simulink model "Microgrid_w_BESS_Q4_1"  (R2024b)
settings: Solver=VariableStepAuto  StartTime=0.0  StopTime=4  RelTol=1e-3
undefined symbols (not defined in the file): DiscIntNeverNeededParam, ini_SoC, Ion, Lithium, Ts, Ts_Control
libraries: simulink x5, ee_lib x5, spsParallelRLCBranchLib x4, nesl_utility x4, spsCurrentVoltageSimscapeInterfaceLib x3, powerlib_extras x3, spsThreePhaseVIMeasurementLib x2, spsSeriesRLCBranchLib x2, spsMultimeterLib x2, spsThreePhaseSeriesRLCBranchLib x2, spsGroundLib x2, slpidlib x2
(part 1 of 2)
settings Model: Creator=DELL  LastModifiedBy=mitphanase
settings DataIOCC: ReturnWorkspaceOutputs=off

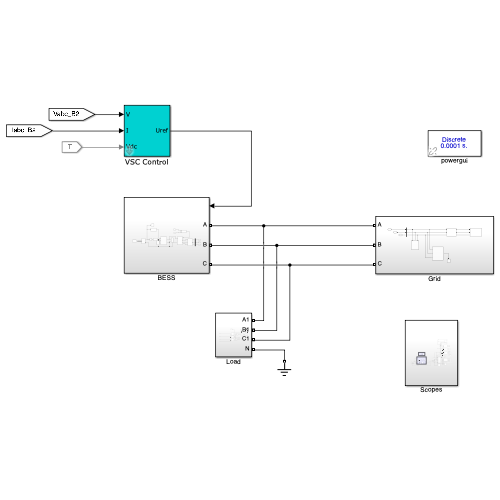
[thumbnail: Simulink's stored preview of the top-level diagram]
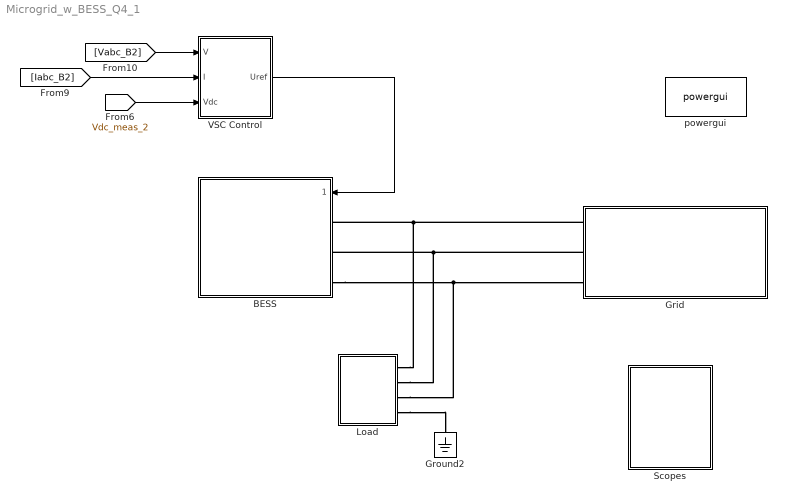
== system Microgrid_w_BESS_Q4_1 ==
  BESS : Subsystem
  Grid : Subsystem
  Ground2 : spsGroundLib/Ground  LConnTagsString=a
  Load : Subsystem
  Scopes : Subsystem
  VSC Control : Subsystem  mask(VSC Main Controller){nom=[10e3  50 ], Vnom=[ 400 400 ], Vnom_dc=600, RLxfo=[0  0 ], RLchoke=[0  0  ], K_VDCreg=[18  600], K_Ireg=[0.2 20], Ts=Ts_Control}
      mask prompts: nom "Nominal power and frequency [ Pnom(VA)  Fnom(Hz) ]:"; Vnom "Nominal primary and secondary voltages (Vrms LL) [ Vnom_prim   Vnom_sec ]:"; Vnom_dc "Nominal DC bus voltage (V):"; RLxfo "Total transformer leakage impedance (pu/Pnom) [ Rxfo  Lxf ]"; RLchoke "Choke impedance [ R(ohm) L(H) ]"; K_VDCreg "VDC regultator gains [ Kp  Ki ]:"; K_Ireg "Current regulator gains [ Kp  Ki ]:"; Ts "Sample time"
      mask init:
      | Pnom=nom(1);
      | Fnom=nom(2);
      | Vnom_prim=Vnom(1);
      | Vnom_sec=Vnom(2);
      | Zbase=Vnom_sec^2/Pnom;
      | Rtot_pu=RLxfo(1) + RLchoke(1)/Zbase;
      | Ltot_pu=RLxfo(2) + RLchoke(2)/(Zbase/(2*pi*Fnom));
      | Kp_VDCreg=K_VDCreg(1);
      | Ki_VDCreg=K_VDCreg(2);
      | Kp_Ireg=K_Ireg(1);
      | Ki_Ireg=K_Ireg(2);
      | Vdc_ref=Vnom_dc;
  powergui : sps_lib/powergui  Priority=1  SimulationMode=Discrete  SampleTime=Ts  frequency=60  Iterations=50  frequencyindice=0  Pbase=100e6  ErrMax=1e-4  UnitsV=kV  UnitsW=MW  buscounter=0  FunctionMessages=off  echomessages=off  EnableUseOfTLC=off  CurrentSourceSwitches=off  DisableSnubberDevices=off  DisableRonSwitches=off  DisableVfSwitches=off  DisplayEquations=off  AutomaticDiscreteSolvers=off  SolverType=Tustin/Backward Euler (TBE)  Interpol=off  ExternalGateDelay=off  methode=off  Ts=100  x0status=blocks  SPID=on  SwTol=0  HookPort=off  NonlinearTolerance=1e-4  nMaxIteration=100  ContinueOnMaxIteration=off  RestoreLinks=warning  ResistiveCurrentMeasurement=off  Frange=[0:2:500]  Ylog=off  Xlog=on  ShowGrid=off  save=off  variable=ZData  structure=0  ZoomFFT=off  StartTime=0.0  cycles=1  DisplayStyle=1  fundamental=60  FreqAxis=off  MaxFrequency=1000  frequencyindicesteady=1  RmsSteady=1  display=off
  wires:
  [Vdc_meas_2] -> VSC Control/3(Vdc)
  [Vabc_B2] -> VSC Control/1(V)
  [Iabc_B2] -> VSC Control/2(I)
  VSC Control/1(Uref) -> BESS/1("  ")
  connections:
  Grid/LConn1 -- Load/LConn1 -- BESS/LConn1
  BESS/LConn3 -- Load/LConn3 -- Grid/LConn3
  Grid/LConn2 -- Load/LConn2 -- BESS/LConn2
  Load/LConn4 -- Ground2/LConn1

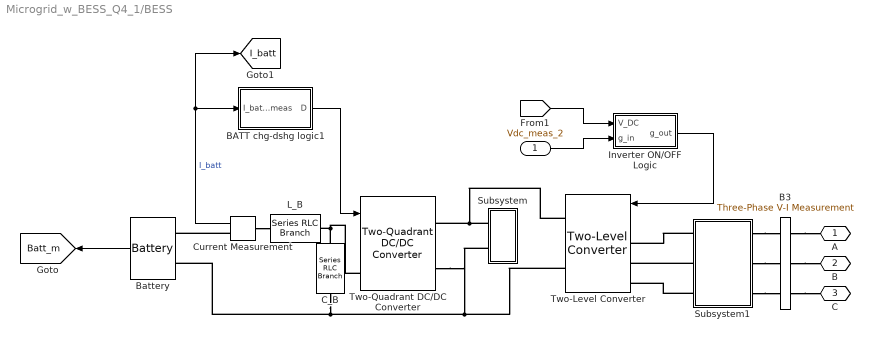
== system Microgrid_w_BESS_Q4_1/BESS ==
  "  " : Inport
  B3 : spsThreePhaseVIMeasurementLib/Three-Phase V-I Measurement  VoltageMeasurement=phase-to-ground  SetLabelV=on  LabelV=Vabc_B3  Vpu=off  VpuLL=off  CurrentMeasurement=yes  SetLabelI=on  LabelI=Iabc_B3  Ipu=off  Pbase=100e6  Vbase=1000  OutputType=Magnitude  PhasorSimulation=off  PSBequivalent=0
  BATT chg-dshg logic1 : Subsystem
  Battery : spsBatteryLib/Battery  BatType=Lithium-Ion  NomV=500  NomQ=20  SOC=ini_SoC  Batt_Tr=0.01  PresetModel=on  MaxQ=20  MinV=375  FullV=581.9936  Dis_rate=8.6957  R=0.25  Normal_OP=18.087  expZone="[540.1929     0.9826087]"
  C_B : spsSeriesRLCBranchLib/Series RLC Branch  LConnTagsString=__new0  RConnTagsString=__new0  BranchType=C  Resistance=10e-3  Inductance=10e-3  SetiL0=off  InitialCurrent=0  Capacitance=100e-6  Setx0=off  InitialVoltage=230  Measurements=None
  Current Measurement : spsCurrentMeasurementLib/Current Measurement  PhasorSimulation=off  OutputType=Complex  PSBequivalent=0
  Inverter ON/OFF Logic : Subsystem
  L_B : spsSeriesRLCBranchLib/Series RLC Branch  LConnTagsString=__new0  RConnTagsString=__new0  BranchType=RL  Resistance=0.5  Inductance=10e-3  SetiL0=off  InitialCurrent=0  Capacitance=100e-6  Setx0=off  InitialVoltage=230  Measurements=None
  Subsystem : Subsystem
  Subsystem1 : Subsystem
  Two-Level Converter : spsTwoLevelConverterLib/Two-Level Converter  ModelType=Average model (Uref-controlled)  Ron=1e-3  Rs=1e6  Cs=inf  Vforward=[0,0]  Ron_Diode=1e-3  Rs_Diode=1e6  Cs_Diode=inf  Vf_Diode=1e-3  Rs_CurrentSource=inf  Ron_ACsource=1e-3
      settings: LibrarySourceBlock=sps_lib/Power Electronics/Two-Level Converter
  Two-Quadrant DC/DC Converter : spsTwoQuadrantDCDCConverterLib/Two-Quadrant DC//DC Converter  ModelType=Average model (D-controlled)  Ron=1e-3  Rs=1e6  Cs=inf  Vforward=[0,0]  Ron_Diode=1e-3  Rs_Diode=1e6  Cs_Diode=inf  Vf_Diode=1e-3  Rs_CurrentSource=inf  Ron_ACsource=1e-3
  A : PMIOPort  Side=Left
  B : PMIOPort  Port=2  Side=Left
  C : PMIOPort  Port=3  Side=Left
  tag scope: Batt_m=global, I_batt=global
  wires:
  BATT chg-dshg logic1/1(D) -> Two-Quadrant DC/DC Converter/1
  [Vdc_meas_2] -> Inverter ON/OFF Logic/1(V_DC)
  "  "/1 -> Inverter ON/OFF Logic/2(g_in)
  Inverter ON/OFF Logic/1(g_out) -> Two-Level Converter/1
  Battery/1 -> [Batt_m]
  Current Measurement/1 -> BATT chg-dshg logic1/1(I_batt_meas), [I_batt]  "I_batt"
  connections:
  Two-Level Converter/RConn2 -- Subsystem/RConn2 -- Two-Quadrant DC/DC Converter/RConn2 -- Battery/LConn2 -- C_B/RConn1
  C_B/LConn1 -- Two-Quadrant DC/DC Converter/LConn1 -- L_B/LConn1
  Subsystem/RConn1 -- Two-Level Converter/RConn1 -- Two-Quadrant DC/DC Converter/RConn1
  Current Measurement/LConn1 -- L_B/RConn1
  Current Measurement/RConn1 -- Battery/LConn1
  B3/RConn1 -- A/RConn1
  B3/RConn2 -- B/RConn1
  B3/RConn3 -- C/RConn1
  Subsystem1/RConn1 -- B3/LConn1
  Subsystem1/RConn2 -- B3/LConn2
  Subsystem1/RConn3 -- B3/LConn3
  Subsystem1/LConn2 -- Two-Level Converter/LConn2
  Subsystem1/LConn1 -- Two-Level Converter/LConn1
  Subsystem1/LConn3 -- Two-Level Converter/LConn3

== system Microgrid_w_BESS_Q4_1/Grid ==
  B2 : spsThreePhaseVIMeasurementLib/Three-Phase V-I Measurement  VoltageMeasurement=phase-to-ground  SetLabelV=on  LabelV=Vabc_B2  Vpu=off  VpuLL=off  CurrentMeasurement=yes  SetLabelI=on  LabelI=Iabc_B2  Ipu=off  Pbase=100e6  Vbase=500e3  OutputType=Magnitude  PhasorSimulation=off  PSBequivalent=0
  Ground : spsGroundLib/Ground  LConnTagsString=a
  "Grounding Transformer " : spsGroundingTransformerLib/Grounding Transformer   UNITS=SI  NominalPower="[3e3   50]"  NominalVoltage=0.4e3  ZeroSequenceImpedance_pu=[0.025 0.75]  MagnetizationBranch_pu=[500 500]  ZeroSequenceImpedance_SI=[1.3333 40]  MagnetizationBranch_SI=[26667 26667]  Measurements=All voltages and currents
      settings: LibrarySourceBlock=|
      | sps_lib/Power Grid Elements/Grounding
      | Transformer
  Three-Phase Series RLC Branch : spsThreePhaseSeriesRLCBranchLib/Three-Phase Series RLC Branch  LConnTagsString=A|B|C  RConnTagsString=A|B|C  BranchType=R  Resistance=1e-3  Inductance=1e-3  Capacitance=1e-6  Measurements=None
  Three-Phase Series RLC Load1 : spsThreePhaseSeriesRLCLoadLib/Three-Phase Series RLC Load  LConnTagsString=A|B|C  Configuration=Y (grounded)  NominalVoltage=400  Vabc=[1e3 1e3 1e3]  Vabcp=[1e3 1e3 1e3]  NominalFrequency=50  UnbalancedPower=off  ActivePower=1  InductivePower=0  CapacitivePower=0  Pabc=[10e3 9e3 11e3]  QLabc=[100 90 110]  QCabc=[100 90 110]  Pabcp=[10e3 9e3 11e3]  QLabcp=[100 90 110]  QCabcp=[100 90 110]  Measurements=None  LoadType=constant Z
  Three-Phase Source : spsThreePhaseSourceLib/Three-Phase Source  InternalConnection=Yg  VoltagePhases=off  Voltage=400  PhaseAngle=0  Voltage_phases=[25e3 25e3 25e3]/sqrt(3)  PhaseAngles_phases=[0 -120 +120]  Frequency=50  NonIdealSource=on  SpecifyImpedance=on  Resistance=0.0113  Inductance=36e-6  ShortCircuitLevel=1e6  BaseVoltage=400  XRratio=4  BusType=swing  Pref=10e3  Qref=0  Prefabc=[10e3, 10e3, 10e3]  Qrefabc=[0, 0, 0]  Qmin=-inf  Qmax=inf
  A : PMIOPort  Side=Left
  B : PMIOPort  Port=2  Side=Left
  C : PMIOPort  Port=3  Side=Left
  connections:
  "Grounding Transformer "/RConn1 -- Ground/LConn1
  B2/LConn1 -- Three-Phase Series RLC Branch/LConn1 -- "Grounding Transformer "/LConn1 -- Three-Phase Series RLC Load1/LConn1
  Three-Phase Series RLC Load1/LConn2 -- Three-Phase Series RLC Branch/LConn2 -- "Grounding Transformer "/LConn2 -- B2/LConn2
  Three-Phase Series RLC Load1/LConn3 -- Three-Phase Series RLC Branch/LConn3 -- "Grounding Transformer "/LConn3 -- B2/LConn3
  B2/RConn3 -- C/RConn1
  B2/RConn2 -- B/RConn1
  B2/RConn1 -- A/RConn1
  Three-Phase Series RLC Branch/RConn1 -- Three-Phase Source/RConn1
  Three-Phase Series RLC Branch/RConn2 -- Three-Phase Source/RConn2
  Three-Phase Series RLC Branch/RConn3 -- Three-Phase Source/RConn3

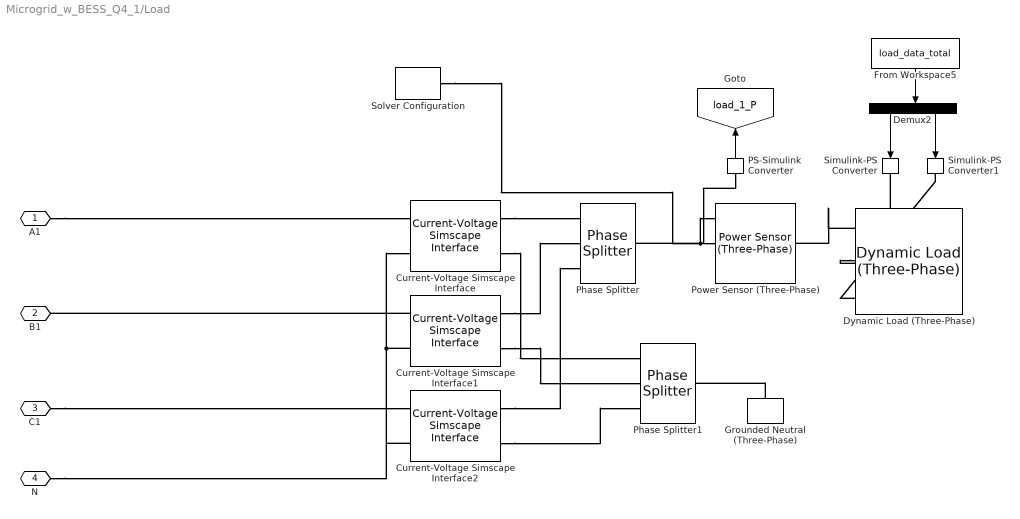
== system Microgrid_w_BESS_Q4_1/Load ==
  Current-Voltage Simscape Interface : spsCurrentVoltageSimscapeInterfaceLib/Current-Voltage Simscape Interface  DFT=off  FMode=Low pass filter (continuous)  T=1e-4  Ts=50e-6  i0=0  v0=0  Sd=Specialized Power Systems side  Measurements=off
  Current-Voltage Simscape Interface1 : spsCurrentVoltageSimscapeInterfaceLib/Current-Voltage Simscape Interface  DFT=off  FMode=Low pass filter (continuous)  T=1e-4  Ts=50e-6  i0=0  v0=0  Sd=Specialized Power Systems side  Measurements=off
  Current-Voltage Simscape Interface2 : spsCurrentVoltageSimscapeInterfaceLib/Current-Voltage Simscape Interface  DFT=off  FMode=Low pass filter (continuous)  T=1e-4  Ts=50e-6  i0=0  v0=0  Sd=Specialized Power Systems side  Measurements=off
  Demux2 : Demux  Outputs=2
  Dynamic Load (Three-Phase) : ee_lib/Passive/Dynamic Load (Three-Phase)  port_option=ee.enum.threePhasePort.composite  FRated=50 Hz  Vline_rms_min=1 V  tau=0.01 s  Vline_rms_ini=400 V  Vang_ini=0 deg  gmin=0 S  fault_action=simscape.enum.assert.action.none  t_fault=1 s
      settings: InternalSimscapePortConfiguration="{\"Bottom\":[],\"Left\":[{\"id\":\"N\",\"label\":\"~\",\"type\":\"foundation.electrical.three_phase\"}],\"Right\":[],\"Top\":[{\"id\":\"P\",\"label\":\"P\",\"type\":\"input\"},{\"id\":\"Q\",\"label\":\"Q\",\"type\":\"input\"}]}"
  From Workspace5 : FromWorkspace  VariableName=load_data_total  SampleTime=0.01
  Grounded Neutral (Three-Phase) : ee_lib/Connectors & References/Grounded Neutral (Three-Phase)
  PS-Simulink Converter : nesl_utility/PS-Simulink Converter  PhysicalDomain=network_engine_domain  SubClassName=ps_output  LeftPortType=input  RightPortType=output  PseudoPeriodic=off  Frequencies=[]  VectorFormat=inherit  Unit=inherit  AffineConversion=off
  Phase Splitter : ee_lib/Connectors & References/Phase Splitter
  Phase Splitter1 : ee_lib/Connectors & References/Phase Splitter
  Power Sensor (Three-Phase) : ee_lib/Sensors & Transducers/Power Sensor (Three-Phase)  load_type=ee.enum.passive.type_balanced.unbalanced  f0=50 Hz  config=ee.enum.with_neutral.no  rho=1
      settings: InternalSimscapePortConfiguration="{\"Bottom\":[],\"Left\":[{\"id\":\"N1\",\"label\":\"~1\",\"type\":\"foundation.electrical.three_phase\"}],\"Right\":[{\"id\":\"N2\",\"label\":\"~2\",\"type\":\"foundation.electrical.three_phase\"}],\"Top\":[{\"id\":\"Pm\",\"label\":\"P\",\"type\":\"output\"},{\"id\":\"Qm\",\"label\":\"Q\",\"type\":\"output\"}]}"
  Simulink-PS Converter : nesl_utility/Simulink-PS Converter  PhysicalDomain=network_engine_domain  SubClassName=ps_input  LeftPortType=input  RightPortType=output  PseudoPeriodic=off  Frequencies=[]  NoiseDistribution=none  NoiseParameters=[]  Unit=1  AffineConversion=off  FilteringAndDerivatives=provide  SimscapeFilterOrder=1  InputFilterTimeConstant=0.001  UdotUserProvided=0
  Simulink-PS Converter1 : nesl_utility/Simulink-PS Converter  PhysicalDomain=network_engine_domain  SubClassName=ps_input  LeftPortType=input  RightPortType=output  PseudoPeriodic=off  Frequencies=[]  NoiseDistribution=none  NoiseParameters=[]  Unit=1  AffineConversion=off  FilteringAndDerivatives=provide  SimscapeFilterOrder=1  InputFilterTimeConstant=0.001  UdotUserProvided=0
  Solver Configuration : nesl_utility/Solver Configuration  PhysicalDomain=network_engine_domain  SubClassName=solver  LeftPortType=input  RightPortType=generic  Tones=[]  Harmonics=[]  SimulateNoise=off  Profile=off  UseLocalSampling=off  EnableSwitchedLinearOptims=on  FrequencyDomain=off  UseCCode=off  RelTol=0.001  AbsTol=0.001  MinStep=1e-09  ToWorkspace=off  RevertToSquareIcSolve=off  NumHomotopyIterations=100  PhasorMode=off  PhasorModeNumHarmonics=1  ConsistencySolver=NEWTON_XTOL_AFTER_FTOL  IndexReductionMethod=DerivativeReplacement  DoDC=on  ResidualTolerance=1e-09  ConsistencyTolSource=GLOBAL  ConsistencyAbsTol=0.001  ConsistencyRelTol=0.001  ConsistencyTolFactor=0.001  UseLocalSolver=off  LocalSolverChoice=NE_BACKWARD_EULER_ADVANCER  ResolveIndetEquations=on  FunctionEvalNumThread=1  LocalSolverSampleTime=0.0001  DoFixedCost=off  MaxNonlinIter=3  MaxModeIter=2  ComputeImpulses=off  ImpulseIterations=2  LinearAlgebra=Sparse  LinearAlgebraNumThread=0  EquationFormulation=NE_TIME_EF  DelaysMemoryBudget=2048  AutomaticFiltering=off  FilteringTimeConstant=0.001  PartitionStorageMethod=AS_NEEDED  PartitionMemoryBudget=1024  PartitionMethod=ROBUST  MultibodyUseLocalSolver=off  MultibodyLocalSolverChoice=ODE1  MultibodyLocalSolverSampleTime=0.001
  A1 : PMIOPort  Side=Left
  B1 : PMIOPort  Port=2  Side=Left
  C1 : PMIOPort  Port=3  Side=Left
  N : PMIOPort  Port=4  Side=Left
  tag scope: load_1_P=global
  wires:
  From Workspace5/1 -> Demux2/1
  Demux2/2 -> Simulink-PS Converter1/1
  PS-Simulink Converter/1 -> [load_1_P]
  Demux2/1 -> Simulink-PS Converter/1
  connections:
  Power Sensor (Three-Phase)/LConn1 -- Solver Configuration/RConn1 -- Phase Splitter/LConn1
  Current-Voltage Simscape Interface1/RConn2 -- Phase Splitter1/RConn2
  Current-Voltage Simscape Interface2/RConn2 -- Phase Splitter1/RConn3
  Dynamic Load (Three-Phase)/LConn1 -- Power Sensor (Three-Phase)/RConn1
  Current-Voltage Simscape Interface1/RConn1 -- Phase Splitter/RConn2
  Current-Voltage Simscape Interface2/RConn1 -- Phase Splitter/RConn3
  Current-Voltage Simscape Interface/RConn1 -- Phase Splitter/RConn1
  Dynamic Load (Three-Phase)/LConn3 -- Simulink-PS Converter1/RConn1
  Grounded Neutral (Three-Phase)/LConn1 -- Phase Splitter1/LConn1
  Current-Voltage Simscape Interface/RConn2 -- Phase Splitter1/RConn1
  PS-Simulink Converter/LConn1 -- Power Sensor (Three-Phase)/LConn2
  Dynamic Load (Three-Phase)/LConn2 -- Simulink-PS Converter/RConn1
  A1/RConn1 -- Current-Voltage Simscape Interface/LConn1
  Current-Voltage Simscape Interface1/LConn1 -- B1/RConn1
  Current-Voltage Simscape Interface1/LConn2 -- N/RConn1 -- Current-Voltage Simscape Interface2/LConn2 -- Current-Voltage Simscape Interface/LConn2
  C1/RConn1 -- Current-Voltage Simscape Interface2/LConn1

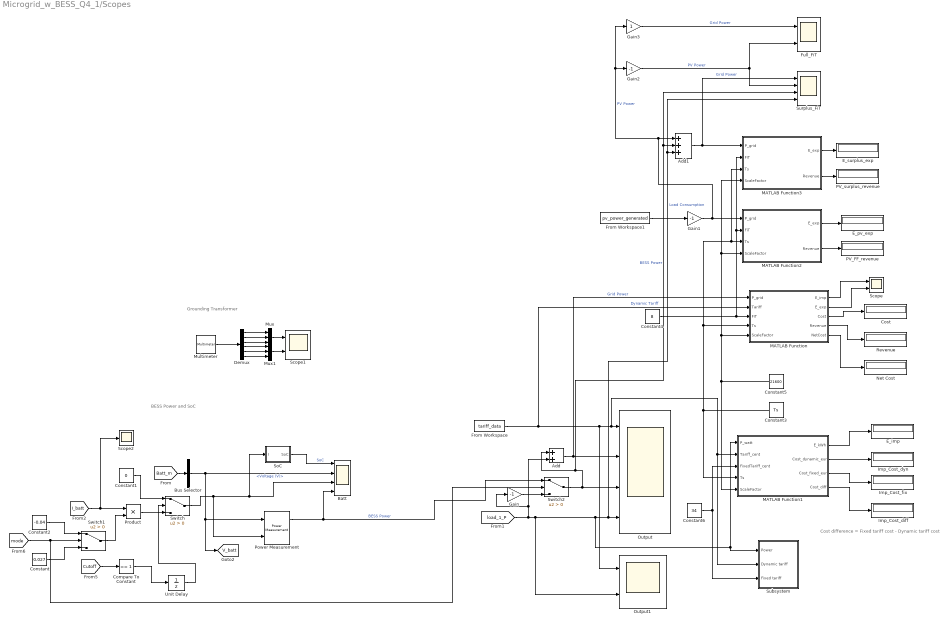
== system Microgrid_w_BESS_Q4_1/Scopes ==
  note: Cost difference = Fixed tariff cost - Dynamic tariff cost
  note: Grounding Transformer
  note: BESS Power and SoC
  Add : Sum
  Add1 : Sum  Inputs=+++
  Batt : Scope  NumInputPorts=4
  Bus Selector : BusSelector  OutputSignals=Voltage (V)
  Compare To Constant : simulink/Logic and Bit Operations/Compare To Constant  relop===  const=1  OutDataTypeStr=uint8
  Constant : Constant  Value=0.027
  Constant1 : Constant  Value=0
  Constant2 : Constant  Value=-0.04
  Constant3 : Constant  Value=Ts
  Constant4 : Constant  Value=8
  Constant5 : Constant  Value=21600
  Constant6 : Constant  Value=34
  Cost : Display
  Demux : Demux  Outputs=6
  E_imp : Display
  E_pv_exp : Display
  E_surplus_exp : Display
  From Workspace : FromWorkspace  VariableName=tariff_data  SampleTime=0.01
  From Workspace1 : FromWorkspace  VariableName=pv_power_generated
  Full_FiT : Scope  NumInputPorts=2
  Gain : Gain  Gain=-1
  Gain1 : Gain  Gain=-1
  Gain2 : Gain  Gain=-1
  Gain3 : Gain
  Imp_Cost_diff : Display
  Imp_Cost_dyn : Display
  Imp_Cost_fix : Display
  MATLAB Function : MATLAB Function  TreatAsAtomicUnit=on
  MATLAB Function1 : MATLAB Function  TreatAsAtomicUnit=on
  MATLAB Function2 : MATLAB Function  TreatAsAtomicUnit=on
  MATLAB Function3 : MATLAB Function  TreatAsAtomicUnit=on
  Multimeter : spsMultimeterLib/Multimeter  L=12  sel=[1 2 3 10 11 12]  yselected={}  Gain=[1 1 1 1 1 1]  OutputType=Complex  PlotAtSimulationStop=off  PhasorSimulation=off
  Mux : Mux  Inputs=3
  Mux1 : Mux  Inputs=3
  Net Cost : Display
  Output : Scope  NumInputPorts=4
  Output1 : Scope  NumInputPorts=2
  PV_FF_revenue : Display
  PV_surplus_revenue : Display
  Power Measurement : eePowerMeasurement/Power Measurement  LabelModeActiveChoice=Discrete  F=50  K=[0]  Ts=Ts_Control
  Product : Product
  Revenue : Display
  Scope : Scope  NumInputPorts=2
  Scope1 : Scope  NumInputPorts=2
  Scope2 : Scope
  SoC : Subsystem
  Subsystem : Subsystem
  Surplus_FiT : Scope  NumInputPorts=4
  Switch : Switch  Criteria=u2 > Threshold  SaturateOnIntegerOverflow=off  InputSameDT=off
  Switch1 : Switch  Criteria=u2 > Threshold  SaturateOnIntegerOverflow=off  InputSameDT=off
  Switch2 : Switch  Criteria=u2 > Threshold  SaturateOnIntegerOverflow=off  InputSameDT=off
  Unit Delay : UnitDelay  SampleTime=-1  HasFrameUpgradeWarning=on
  tag scope: V_batt=global
  wires:
  SoC/1(SoC) -> Batt/1  "SoC"
  [Batt_m] -> Bus Selector/1
  [load_1_P] -> Add/2, Gain/1, Output1/2, MATLAB Function1/1(P_watt), Subsystem/1(Power), Add1/3, Surplus_FiT/4, Output/4  "Load Consumption"
  Multimeter/1 -> Demux/1
  Demux/1 -> Mux/1
  Demux/2 -> Mux/2
  Mux/1 -> Scope1/1
  Demux/3 -> Mux/3
  Demux/4 -> Mux1/1
  Demux/5 -> Mux1/2
  Demux/6 -> Mux1/3
  Mux1/1 -> Scope1/2
  Bus Selector/1 -> Batt/2, Power Measurement/1, [V_batt]  "<Voltage (V)>"
  [I_batt] -> Scope2/1, Product/1
  Switch/1 -> SoC/1(I), Batt/3, Power Measurement/2
  [Cutoff] -> Compare To Constant/1
  Product/1 -> Switch/3
  Constant1/1 -> Switch/1
  Constant2/1 -> Switch1/1
  Constant/1 -> Switch1/3
  Switch1/1 -> Product/2
  [mode] -> Switch2/2, Switch1/2
  Compare To Constant/1 -> Unit Delay/1
  Unit Delay/1 -> Switch/2
  Power Measurement/1 -> Batt/4, Switch2/1  "BESS Power"
  From Workspace/1 -> MATLAB Function/2(Tariff), Output1/1, Subsystem/2(Dynamic tariff), MATLAB Function1/2(Tariff_cent), Output/1  "Dynamic Tariff"
  Add/1 -> MATLAB Function/1(P_grid), Output/2  "Grid Power"
  Constant3/1 -> MATLAB Function3/3(Ts), MATLAB Function2/3(Ts), MATLAB Function/4(Ts), MATLAB Function1/4(Ts)
  MATLAB Function/3(Cost) -> Cost/1
  MATLAB Function/1(E_imp) -> Scope/1
  MATLAB Function/2(E_exp) -> Scope/2
  Constant4/1 -> MATLAB Function3/2(FiT), MATLAB Function2/2(FiT), MATLAB Function/3(FiT)
  MATLAB Function/4(Revenue) -> Revenue/1
  MATLAB Function/5(NetCost) -> Net Cost/1
  Switch2/1 -> Add1/2, Surplus_FiT/3, Add/1, Output/3  "BESS Power"
  Gain/1 -> Switch2/3
  Constant5/1 -> MATLAB Function1/5(ScaleFactor), MATLAB Function3/4(ScaleFactor), MATLAB Function2/4(ScaleFactor), MATLAB Function/5(ScaleFactor)
  MATLAB Function1/1(E_kWh) -> E_imp/1
  MATLAB Function1/2(Cost_dynamic_eur) -> Imp_Cost_dyn/1
  Constant6/1 -> Subsystem/3(Fixed tariff), MATLAB Function1/3(FixedTariff_cent)
  MATLAB Function1/4(Cost_diff) -> Imp_Cost_diff/1
  MATLAB Function1/3(Cost_fixed_eur) -> Imp_Cost_fix/1
  MATLAB Function2/1(E_exp) -> E_pv_exp/1
  MATLAB Function2/2(Revenue) -> PV_FF_revenue/1
  Gain1/1 -> Gain3/1, Gain2/1, Add1/1, MATLAB Function2/1(P_grid)  "PV Power"
  From Workspace1/1 -> Gain1/1
  Add1/1 -> Surplus_FiT/1, MATLAB Function3/1(P_grid)  "Grid Power"
  MATLAB Function3/1(E_exp) -> E_surplus_exp/1
  MATLAB Function3/2(Revenue) -> PV_surplus_revenue/1
  Gain2/1 -> Full_FiT/2, Surplus_FiT/2  "PV Power"
  Gain3/1 -> Full_FiT/1  "Grid Power"

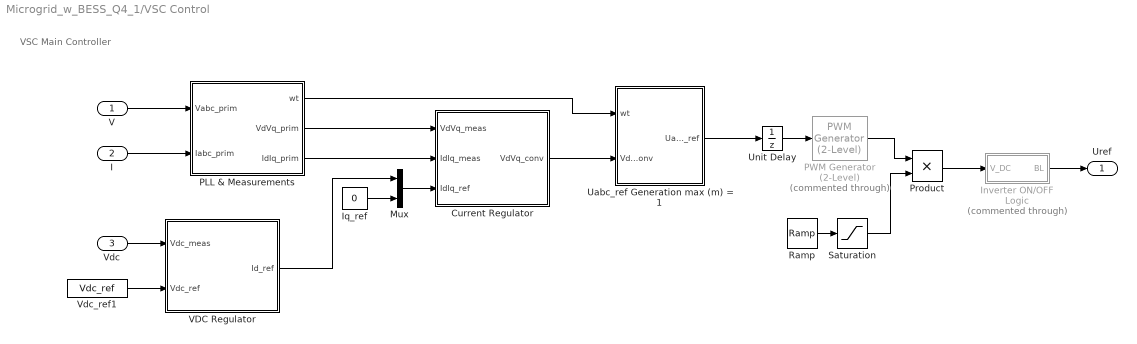
== system Microgrid_w_BESS_Q4_1/VSC Control ==
  note: VSC Main Controller
  V : Inport  PortDimensions=3
  I : Inport  Port=2  PortDimensions=3
  Vdc : Inport  Port=3  PortDimensions=1
  Current Regulator : Subsystem
  Inverter ON/OFF Logic : Subsystem  Commented=through
  Iq_ref : Constant  Value=0
  Mux : Mux  Inputs=2
  PLL & Measurements : Subsystem
  PWM Generator (2-Level) : spsPWMGenerator2LevelLib/PWM Generator (2-Level)  Commented=through  ModulatorType=Three-phase bridge (6 pulses)  ModulatorMode=Unsynchronized  Fc=27*50*8  Pc=90  nF=27  MinMax="[ -1  1 ]"  SamplingTechnique=Natural  ModulatingSignals=off  m=0.8  Freq=60  Phase=0  Ts=Ts_Control  ShowCarrierOutport=off
  Product : Product
  Ramp : simulink/Sources/Ramp  slope=1/0.02  start=0  InitialOutput=0
  Saturation : Saturate  UpperLimit=1  LowerLimit=0
  Uabc_ref Generation max (m) = 1 : Subsystem
  Unit Delay : UnitDelay  SampleTime=Ts_Control  HasFrameUpgradeWarning=on
  VDC Regulator : Subsystem
  Vdc_ref1 : Constant  Value=Vdc_ref
  Uref : Outport  VectorParamsAs1DForOutWhenUnconnected=off
  wires:
  Vdc_ref1/1 -> VDC Regulator/2(Vdc_ref)
  Uabc_ref Generation max (m) = 1/1(Uabc_ref) -> Unit Delay/1
  Unit Delay/1 -> PWM Generator (2-Level)/1
  I/1 -> PLL & Measurements/2(Iabc_prim)
  V/1 -> PLL & Measurements/1(Vabc_prim)
  Vdc/1 -> VDC Regulator/1(Vdc_meas)
  PLL & Measurements/2(VdVq_prim) -> Current Regulator/1(VdVq_meas)
  PLL & Measurements/3(IdIq_prim) -> Current Regulator/2(IdIq_meas)
  Mux/1 -> Current Regulator/3(IdIq_ref)
  Iq_ref/1 -> Mux/2
  PLL & Measurements/1(wt) -> Uabc_ref Generation max (m) = 1/1(wt)
  VDC Regulator/1(Id_ref) -> Mux/1
  PWM Generator (2-Level)/1 -> Product/1
  Current Regulator/1(VdVq_conv) -> Uabc_ref Generation max (m) = 1/2(VdVq_conv)
  Product/1 -> Inverter ON/OFF Logic/1(V_DC)
  Ramp/1 -> Saturation/1
  Saturation/1 -> Product/2
  Inverter ON/OFF Logic/1(BL) -> Uref/1

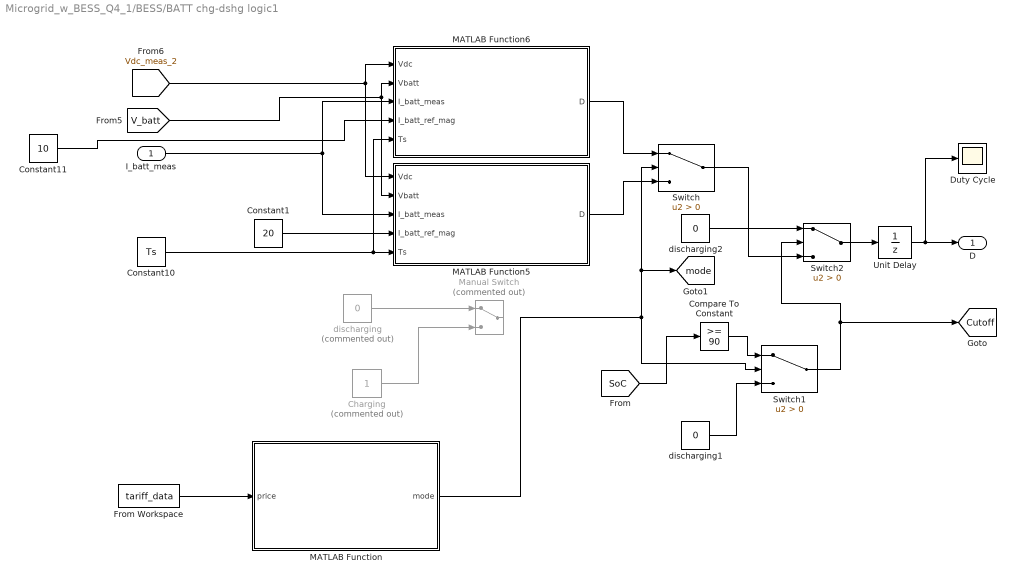
== system Microgrid_w_BESS_Q4_1/BESS/BATT chg-dshg logic1 ==
  I_batt_meas : Inport
  Charging : Constant  Commented=on
  Compare To Constant : simulink/Logic and Bit Operations/Compare To Constant  relop=>=  const=90  OutDataTypeStr=boolean
  Constant1 : Constant  Value=20
  Constant10 : Constant  Value=Ts
  Constant11 : Constant  Value=10
  Duty Cycle : Scope
  From Workspace : FromWorkspace  VariableName=tariff_data  SampleTime=0.01
  MATLAB Function : MATLAB Function  TreatAsAtomicUnit=on
  MATLAB Function5 : MATLAB Function  TreatAsAtomicUnit=on
  MATLAB Function6 : MATLAB Function  TreatAsAtomicUnit=on
  Manual Switch : ManualSwitch  Commented=on
  Switch : Switch  Criteria=u2 > Threshold  SaturateOnIntegerOverflow=off  InputSameDT=off
  Switch1 : Switch  Criteria=u2 > Threshold  SaturateOnIntegerOverflow=off  InputSameDT=off
  Switch2 : Switch  Criteria=u2 > Threshold  SaturateOnIntegerOverflow=off  InputSameDT=off
  Unit Delay : UnitDelay  SampleTime=-1  HasFrameUpgradeWarning=on
  discharging : Constant  Commented=on  Value=0
  discharging1 : Constant  Value=0
  discharging2 : Constant  Value=0
  D : Outport
  tag scope: Cutoff=global, mode=global
  wires:
  Unit Delay/1 -> Duty Cycle/1, D/1
  I_batt_meas/1 -> MATLAB Function6/3(I_batt_meas), MATLAB Function5/3(I_batt_meas)
  [V_batt] -> MATLAB Function5/2(Vbatt), MATLAB Function6/2(Vbatt)
  [Vdc_meas_2] -> MATLAB Function5/1(Vdc), MATLAB Function6/1(Vdc)
  Constant11/1 -> MATLAB Function6/4(I_batt_ref_mag)
  Constant10/1 -> MATLAB Function6/5(Ts), MATLAB Function5/5(Ts)
  MATLAB Function6/1(D) -> Switch/1
  MATLAB Function5/1(D) -> Switch/3
  discharging/1 -> Manual Switch/1
  Charging/1 -> Manual Switch/2
  MATLAB Function/1(mode) -> Switch1/2, Switch/2, [mode]
  Constant1/1 -> MATLAB Function5/4(I_batt_ref_mag)
  [SoC] -> Compare To Constant/1
  Compare To Constant/1 -> Switch1/1
  Switch2/1 -> Unit Delay/1
  Switch/1 -> Switch2/3
  discharging2/1 -> Switch2/1
  discharging1/1 -> Switch1/3
  Switch1/1 -> [Cutoff], Switch2/2
  From Workspace/1 -> MATLAB Function/1(price)

== system Microgrid_w_BESS_Q4_1/BESS/Inverter ON//OFF Logic ==
  V_DC : Inport
  g_in : Inport  Port=2
  Compare To Constant : simulink/Logic and Bit Operations/Compare To Constant  relop=>  const=700  OutDataTypeStr=boolean
  Data Type Conversion : DataTypeConversion  OutDataTypeStr=double  SaturateOnIntegerOverflow=off  RndMeth=Floor
  Product : Product
  Unit Delay : UnitDelay  SampleTime=-1  HasFrameUpgradeWarning=on
  g_out : Outport
  wires:
  Data Type Conversion/1 -> Product/1
  V_DC/1 -> Compare To Constant/1
  Compare To Constant/1 -> Data Type Conversion/1
  Product/1 -> Unit Delay/1
  g_in/1 -> Product/2
  Unit Delay/1 -> g_out/1

== system Microgrid_w_BESS_Q4_1/BESS/Subsystem ==
  C_out_1 : spsParallelRLCBranchLib/Parallel RLC Branch  LConnTagsString=a  RConnTagsString=__new0  BranchType=RC  Resistance=20  Inductance=1e-3  SetiL0=off  InitialCurrent=0  Capacitance=2000e-6  Setx0=off  InitialVoltage=700  Measurements=None
  Voltage Measurement : spsVoltageMeasurementLib/Voltage Measurement  PhasorSimulation=off  OutputType=Complex  PSBequivalent=0
  + : PMIOPort  Side=Right
  - : PMIOPort  Port=2  Side=Right
  tag scope: Vdc_meas_2=global
  wires:
  Voltage Measurement/1 -> [Vdc_meas_2]
  connections:
  Voltage Measurement/LConn2 -- C_out_1/RConn1 -- -/RConn1
  Voltage Measurement/LConn1 -- C_out_1/LConn1 -- +/RConn1

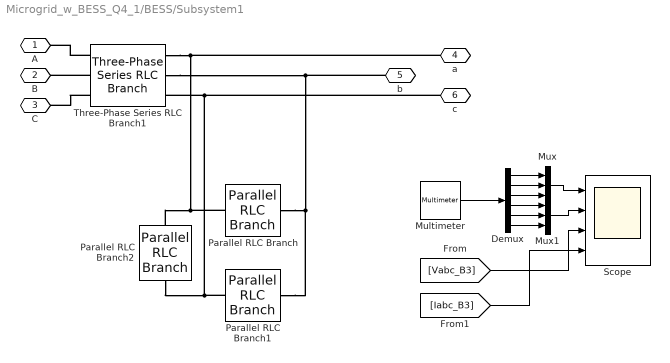
== system Microgrid_w_BESS_Q4_1/BESS/Subsystem1 ==
  Demux : Demux  Outputs=6
  Multimeter : spsMultimeterLib/Multimeter  L=12  sel=[4 5 6 7 8 9]  yselected={}  Gain=[1 1 1 1 1 1]  OutputType=Complex  PlotAtSimulationStop=off  PhasorSimulation=off
  Mux : Mux  Inputs=3
  Mux1 : Mux  Inputs=3
  Parallel RLC Branch : spsParallelRLCBranchLib/Parallel RLC Branch  LConnTagsString=a  RConnTagsString=__new0  BranchType=RC  Resistance=10  Inductance=1e-3  SetiL0=off  InitialCurrent=0  Capacitance=2*1.32e-6  Setx0=off  InitialVoltage=0  Measurements=Branch current
  Parallel RLC Branch1 : spsParallelRLCBranchLib/Parallel RLC Branch  LConnTagsString=a  RConnTagsString=__new0  BranchType=RC  Resistance=10  Inductance=1e-3  SetiL0=off  InitialCurrent=0  Capacitance=2*1.32e-6  Setx0=off  InitialVoltage=0  Measurements=Branch current
  Parallel RLC Branch2 : spsParallelRLCBranchLib/Parallel RLC Branch  LConnTagsString=a  RConnTagsString=__new0  BranchType=RC  Resistance=10  Inductance=1e-3  SetiL0=off  InitialCurrent=0  Capacitance=2*1.32e-6  Setx0=off  InitialVoltage=0  Measurements=Branch current
  Scope : Scope  NumInputPorts=4
  Three-Phase Series RLC Branch1 : spsThreePhaseSeriesRLCBranchLib/Three-Phase Series RLC Branch  LConnTagsString=A|B|C  RConnTagsString=A|B|C  BranchType=L  Resistance=1  Inductance=50e-3  Capacitance=1e-6  Measurements=Branch currents
  A : PMIOPort  Side=Left
  B : PMIOPort  Port=2  Side=Left
  C : PMIOPort  Port=3  Side=Left
  a : PMIOPort  Port=4  Side=Right
  b : PMIOPort  Port=5  Side=Right
  c : PMIOPort  Port=6  Side=Right
  wires:
  [Iabc_B3] -> Scope/4
  [Vabc_B3] -> Scope/3
  Mux1/1 -> Scope/2
  Demux/6 -> Mux1/3
  Demux/5 -> Mux1/2
  Demux/4 -> Mux1/1
  Mux/1 -> Scope/1
  Demux/3 -> Mux/3
  Demux/2 -> Mux/2
  Demux/1 -> Mux/1
  Multimeter/1 -> Demux/1
  connections:
  Parallel RLC Branch/RConn1 -- Parallel RLC Branch1/LConn1 -- b/RConn1 -- Three-Phase Series RLC Branch1/RConn2
  Parallel RLC Branch/LConn1 -- Parallel RLC Branch2/RConn1 -- a/RConn1 -- Three-Phase Series RLC Branch1/RConn1
  Three-Phase Series RLC Branch1/LConn1 -- A/RConn1
  Three-Phase Series RLC Branch1/LConn2 -- B/RConn1
  Three-Phase Series RLC Branch1/LConn3 -- C/RConn1
  Three-Phase Series RLC Branch1/RConn3 -- c/RConn1 -- Parallel RLC Branch1/RConn1 -- Parallel RLC Branch2/LConn1

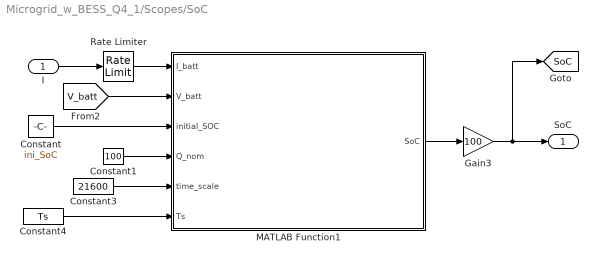
== system Microgrid_w_BESS_Q4_1/Scopes/SoC ==
  I : Inport
  Constant : Constant  Value=ini_SoC
  Constant1 : Constant  Value=100
  Constant3 : Constant  Value=21600
  Constant4 : Constant  Value=Ts
  Gain3 : Gain  Gain=100
  MATLAB Function1 : MATLAB Function  TreatAsAtomicUnit=on
  Rate Limiter : RateLimiter  RisingSlewLimit=500  FallingSlewLimit=-100  SampleTimeMode=inherited
  SoC : Outport
  tag scope: SoC=global
  wires:
  MATLAB Function1/1(SoC) -> Gain3/1
  [V_batt] -> MATLAB Function1/2(V_batt)
  Constant/1 -> MATLAB Function1/3(initial_SOC)
  Constant1/1 -> MATLAB Function1/4(Q_nom)
  Constant3/1 -> MATLAB Function1/5(time_scale)
  Constant4/1 -> MATLAB Function1/6(Ts)
  I/1 -> Rate Limiter/1
  Gain3/1 -> [SoC], SoC/1
  Rate Limiter/1 -> MATLAB Function1/1(I_batt)

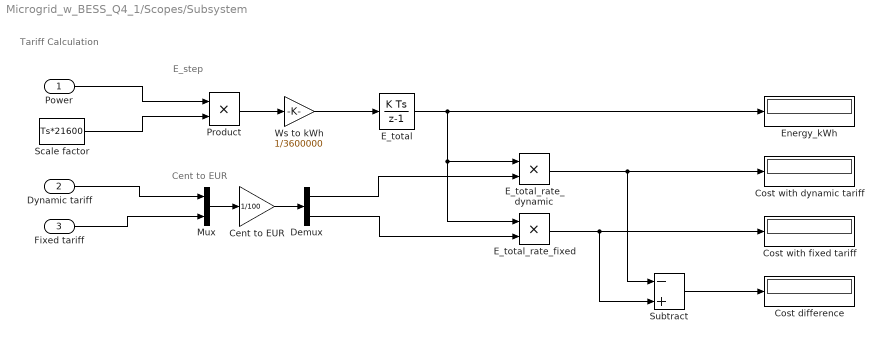
== system Microgrid_w_BESS_Q4_1/Scopes/Subsystem ==
  note: Cent to EUR
  note: Tariff Calculation
  note: E_step
  Power : Inport
  Dynamic tariff : Inport  Port=2
  Fixed tariff : Inport  Port=3
  Cent to EUR : Gain  Gain=1/100
  Cost difference : Display
  Cost with dynamic tariff : Display
  Cost with fixed tariff : Display
  Demux : Demux  Outputs=2
  E_total : DiscreteIntegrator  gainval=10000  SampleTime=-1  ICPrevOutput=DiscIntNeverNeededParam  ICPrevScaledInput=DiscIntNeverNeededParam
  E_total_rate_dynamic : Product
  E_total_rate_fixed : Product
  Energy_kWh : Display
  Mux : Mux  Inputs=2
  Product : Product
  Scale factor : Constant  Value=Ts*21600
  Subtract : Sum  Inputs=-+
  Ws to kWh : Gain  Gain=1/3600000
  wires:
  Power/1 -> Product/1
  Scale factor/1 -> Product/2
  Product/1 -> Ws to kWh/1
  Fixed tariff/1 -> Mux/2
  Dynamic tariff/1 -> Mux/1
  Mux/1 -> Cent to EUR/1
  Ws to kWh/1 -> E_total/1
  Cent to EUR/1 -> Demux/1
  Demux/1 -> E_total_rate_dynamic/2
  Demux/2 -> E_total_rate_fixed/2
  E_total_rate_fixed/1 -> Subtract/2, Cost with fixed tariff/1
  E_total_rate_dynamic/1 -> Subtract/1, Cost with dynamic tariff/1
  E_total/1 -> Energy_kWh/1, E_total_rate_fixed/1, E_total_rate_dynamic/1
  Subtract/1 -> Cost difference/1

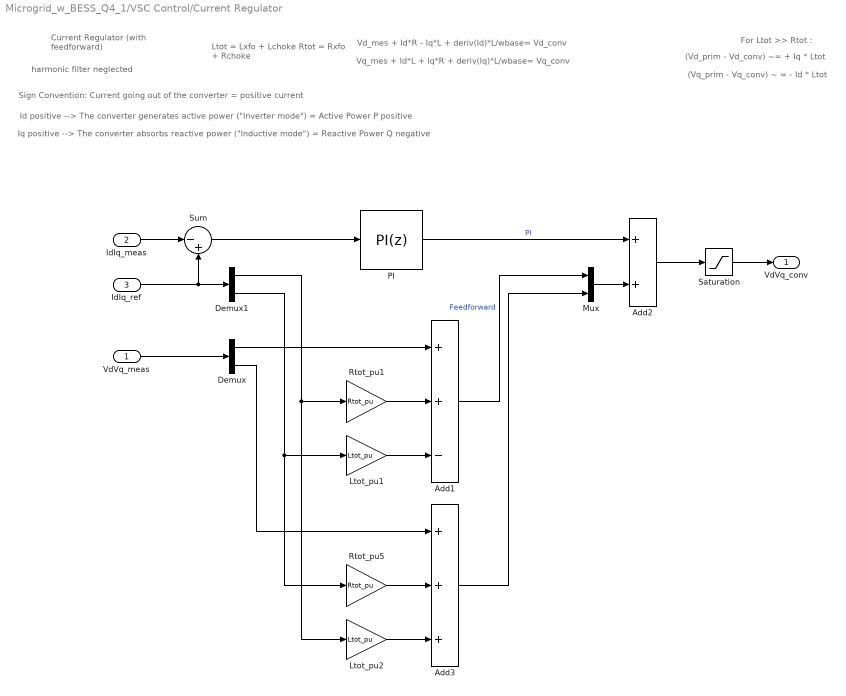
== system Microgrid_w_BESS_Q4_1/VSC Control/Current Regulator ==
  note: For Ltot >> Rtot :
  note: (Vq_prim - Vq_conv) ~ = - Id * Ltot
  note: (Vd_prim - Vd_conv) ~= + Iq * Ltot
  note: Ltot = Lxfo + Lchoke
      | Rtot = Rxfo + Rchoke
  note: Id positive --> The converter generates active power ("Inverter mode") = Active Power P positive
  note: Iq positive --> The converter absorbs reactive power ("Inductive mode") = Reactive Power Q negative
  note: Sign Convention: Current going out of the converter = positive current
  note: Current Regulator
      | (with feedforward)
  note: Vq_mes + Id*L + Iq*R + deriv(Iq)*L/wbase= Vq_conv
  note: Vd_mes + Id*R - Iq*L + deriv(Id)*L/wbase= Vd_conv
  note: harmonic filter neglected
  VdVq_meas : Inport  PortDimensions=2
  IdIq_meas : Inport  Port=2  PortDimensions=2
  IdIq_ref : Inport  Port=3  PortDimensions=2
  Add1 : Sum  Inputs=++-
  Add2 : Sum
  Add3 : Sum  Inputs=+++
  Demux : Demux  Outputs=2
  Demux1 : Demux  Outputs=2
  Ltot_pu1 : Gain  Gain=Ltot_pu  SaturateOnIntegerOverflow=on  OutDataTypeStr=Inherit: Same as input  ParamDataTypeStr=Inherit: Same as input
  Ltot_pu2 : Gain  Gain=Ltot_pu  SaturateOnIntegerOverflow=on  OutDataTypeStr=Inherit: Same as input  ParamDataTypeStr=Inherit: Same as input
  Mux : Mux  Inputs=2
  PI : slpidlib/PID Controller  Controller=PI  Form=Parallel  TimeDomain=Discrete-time  UseExternalTs=off  SampleTime=Ts  IntegratorMethod=Forward Euler  FilterMethod=Forward Euler  ControllerParametersSource=internal  P=Kp_Ireg  I=Ki_Ireg  UseKiTs=off  D=0  UseExternalDerivativeSource=off  N=100  UseFilter=on  TunerSelectOption=Transfer Function Based (PID Tuner App)  InitialConditionSource=internal  InitialConditionForIntegrator=0  InitialConditionForFilter=0  DifferentiatorICPrevScaledInput=0  ExternalReset=none  TrackingMode=off  Kt=1  LimitOutput=on  SatLimitsSource=internal  UpperSaturationLimit=2  LowerSaturationLimit=-2  LinearizeAsGain=off  AntiWindupMode=none  Kb=1  LimitIntegrator=off  UpperIntegratorSaturationLimit=inf  LowerIntegratorSaturationLimit=-inf  POutMin=[]  POutMax=[]  IOutMin=[]  IOutMax=[]  DOutMin=[]  DOutMax=[]  NOutMin=[]  NOutMax=[]  SumOutMin=[]  SumOutMax=[]  SaturationOutMin=[]  SaturationOutMax=[]  PParamMin=[]  PParamMax=[]  IParamMin=[]  IParamMax=[]  DParamMin=[]  DParamMax=[]  NParamMin=[]  NParamMax=[]  KbParamMin=[]  KbParamMax=[]  KtParamMin=[]  KtParamMax=[]  KbOutMin=[]  KbOutMax=[]  KtOutMin=[]  KtOutMax=[]  IntegratorOutMin=[]  IntegratorOutMax=[]  FilterOutMin=[]  FilterOutMax=[]  SumI1OutMin=[]  SumI1OutMax=[]  SumI2OutMin=[]  SumI2OutMax=[]  SumI3OutMin=[]  SumI3OutMax=[]  SumI4OutMin=[]  SumI4OutMax=[]  SumDOutMin=[]  SumDOutMax=[]  DifferentiatorOutMin=[]  DifferentiatorOutMax=[]  FilterDiffOutCoefMin=[]  FilterDiffOutCoefMax=[]  ReciprocalOutMin=[]  ReciprocalOutMax=[]  SumDenOutMin=[]  SumDenOutMax=[]  SumNumOutMin=[]  SumNumOutMax=[]  DivideOutMin=[]  DivideOutMax=[]  UdiffTsProdOutMin=[]  UdiffTsProdOutMax=[]  NTsProdOutMin=[]  NTsProdOutMax=[]  UintegralTsProdOutMin=[]  UintegralTsProdOutMax=[]  UngainTsProdOutMin=[]  UngainTsProdOutMax=[]  ClampingZeroOutDataTypeStr=Inherit: Inherit via back propagation  ClampingZeroOutMin=[]  ClampingZeroOutMax=[]  FilterDenConstantOutDataTypeStr=Inherit: Inherit via back propagation  FilterDenConstantOutMin=[]  FilterDenConstantOutMax=[]  PCopyOutDataTypeStr=Inherit: Inherit via back propagation  PCopyOutMin=[]  PCopyOutMax=[]  NCopyOutDataTypeStr=Inherit: Inherit via back propagation  NCopyOutMin=[]  NCopyOutMax=[]  IntegratorContinuousStateAttributes=''  IntegratorStateMustResolveToSignalObject=off  IntegratorRTWStateStorageClass=Auto  FilterContinuousStateAttributes=''  FilterStateMustResolveToSignalObject=off  FilterRTWStateStorageClass=Auto  ParallelPVariant=InternalParameters  IdealPVariant=Disabled  IVariant=InternalParameters  DVariant=Disabled  IntegratorVariant=Discrete  SatVariant=Enabled  AWVariant=Passthrough  PCopyVariant=Disabled  TRVariant=Disabled  FdbkBlocksVariant=Forward  IdealPFdbkVariant=Disabled  SatFdbkVariant=Disabled  DerivativeFilterVariant=Disabled  NVariant=Disabled  NCopyVariant=Disabled_SignalSpec  FilterICVariant=Disabled  IntegratorICVariant=InternalICs  ExternalResetVariant=Disabled  TRSumVariant=Passthrough  SumFdbkVariant=Disabled  SumVariant=Sum_PI  TsampFilterVariant=InternalTs  TsampNgainVariant=Passthrough  TsampIntegralVariant=Disabled_SignalSpec  ExternalSaturationOutDataTypeStr=Inherit: Same as second input  DerivativeSourceVariant=Disabled  PreIntVariant=InternalPreInt
  Rtot_pu1 : Gain  Gain=Rtot_pu  SaturateOnIntegerOverflow=on  OutDataTypeStr=Inherit: Same as input  ParamDataTypeStr=Inherit: Same as input
  Rtot_pu5 : Gain  Gain=Rtot_pu  SaturateOnIntegerOverflow=on  OutDataTypeStr=Inherit: Same as input  ParamDataTypeStr=Inherit: Same as input
  Saturation : Saturate  UpperLimit=2  LowerLimit=-2
  Sum : Sum  Inputs=|-+
  VdVq_conv : Outport  VectorParamsAs1DForOutWhenUnconnected=off
  wires:
  Add3/1 -> Mux/2
  Demux/2 -> Add3/1
  Add1/1 -> Mux/1  "Feedforward"
  Ltot_pu2/1 -> Add3/3
  Rtot_pu5/1 -> Add3/2
  Demux1/2 -> Rtot_pu5/1, Ltot_pu1/1
  Ltot_pu1/1 -> Add1/3
  Demux1/1 -> Ltot_pu2/1, Rtot_pu1/1
  Rtot_pu1/1 -> Add1/2
  Demux/1 -> Add1/1
  VdVq_meas/1 -> Demux/1
  Saturation/1 -> VdVq_conv/1
  Add2/1 -> Saturation/1
  IdIq_meas/1 -> Sum/1
  IdIq_ref/1 -> Demux1/1, Sum/2
  Sum/1 -> PI/1
  PI/1 -> Add2/1  "PI"
  Mux/1 -> Add2/2

== system Microgrid_w_BESS_Q4_1/VSC Control/Inverter ON//OFF Logic ==
  V_DC : Inport
  AND : Logic  Operator=NAND  IconShape=distinctive  AllPortsSameDT=off  OutDataTypeStr=boolean
  Compare To Constant : simulink/Logic and Bit Operations/Compare To Constant  relop=>=  const=200  OutDataTypeStr=boolean
  Constant : Constant
  Data Type Conversion : DataTypeConversion  OutDataTypeStr=double  SaturateOnIntegerOverflow=off  RndMeth=Floor
  BL : Outport
  tag scope: inv_cont_1=global
  wires:
  Data Type Conversion/1 -> [inv_cont_1], BL/1
  V_DC/1 -> Compare To Constant/1
  AND/1 -> Data Type Conversion/1
  Compare To Constant/1 -> AND/1
  Constant/1 -> AND/2

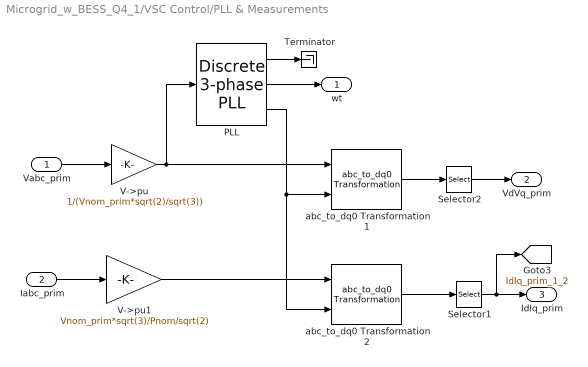
== system Microgrid_w_BESS_Q4_1/VSC Control/PLL & Measurements ==
  Vabc_prim : Inport
  Iabc_prim : Inport  Port=2
  PLL : powerlib_extras/Discrete  Control Blocks/Discrete 3-phase PLL  Fmin=45  Par_Init="[-0.57  Fnom]"  ParK=[60 1400]  Ts=Ts  AGC=off
  Selector1 : Selector  InputPortWidth=3  IndexOptions=Index vector (dialog)  Indices=[1 2]  OutputSizes=1
  Selector2 : Selector  InputPortWidth=3  IndexOptions=Index vector (dialog)  Indices=[1 2]  OutputSizes=1
  Terminator : Terminator
  V->pu : Gain  Gain=1/(Vnom_prim*sqrt(2)/sqrt(3))  SaturateOnIntegerOverflow=on  OutDataTypeStr=Inherit: Same as input  ParamDataTypeStr=Inherit: Same as input
  V->pu1 : Gain  Gain=Vnom_prim*sqrt(3)/Pnom/sqrt(2)  SaturateOnIntegerOverflow=on  OutDataTypeStr=Inherit: Same as input  ParamDataTypeStr=Inherit: Same as input
  abc_to_dq0 Transformation1 : powerlib_extras/Measurements/abc_to_dq0 Transformation
  abc_to_dq0 Transformation2 : powerlib_extras/Measurements/abc_to_dq0 Transformation
  wt : Outport  VectorParamsAs1DForOutWhenUnconnected=off
  VdVq_prim : Outport  Port=2  VectorParamsAs1DForOutWhenUnconnected=off
  IdIq_prim : Outport  Port=3  VectorParamsAs1DForOutWhenUnconnected=off
  tag scope: IdIq_prim_1_2=global
  wires:
  PLL/1 -> Terminator/1
  PLL/3 -> abc_to_dq0 Transformation1/2, abc_to_dq0 Transformation2/2
  Selector1/1 -> IdIq_prim/1, [IdIq_prim_1_2]
  Selector2/1 -> VdVq_prim/1
  abc_to_dq0 Transformation1/1 -> Selector2/1
  Iabc_prim/1 -> V->pu1/1
  Vabc_prim/1 -> V->pu/1
  PLL/2 -> wt/1
  abc_to_dq0 Transformation2/1 -> Selector1/1
  V->pu/1 -> abc_to_dq0 Transformation1/1, PLL/1
  V->pu1/1 -> abc_to_dq0 Transformation2/1

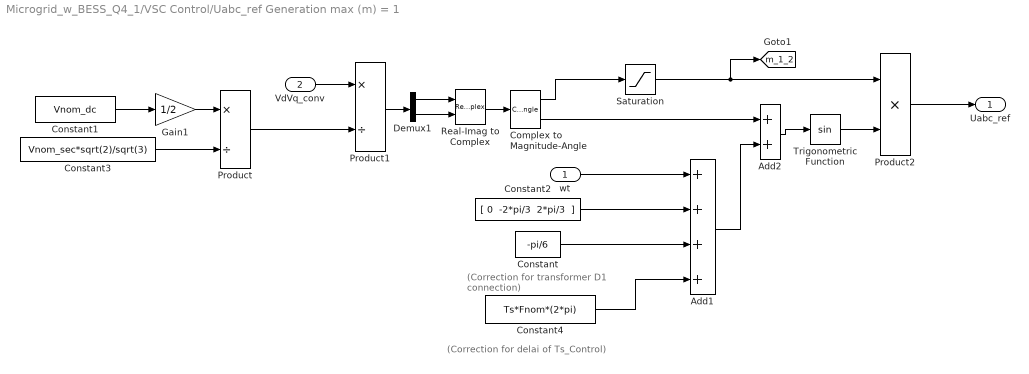
== system Microgrid_w_BESS_Q4_1/VSC Control/Uabc_ref Generation max (m) = 1 ==
  note: (Correction for delai of Ts_Control)
  note: (Correction for transformer
      |  D1 connection)
  wt : Inport
  VdVq_conv : Inport  Port=2
  Add1 : Sum  Inputs=++++
  Add2 : Sum
  Complex to Magnitude-Angle : ComplexToMagnitudeAngle
  Constant : Constant  Value=-pi/6
  Constant1 : Constant  Value=Vnom_dc
  Constant2 : Constant  Value="[ 0  -2*pi/3  2*pi/3  ]"
  Constant3 : Constant  Value=Vnom_sec*sqrt(2)/sqrt(3)
  Constant4 : Constant  Value=Ts*Fnom*(2*pi)
  Demux1 : Demux  Outputs=2
  Gain1 : Gain  Gain=1/2
  Product : Product  Inputs=*/  RndMeth=Zero
  Product1 : Product  Inputs=*/  RndMeth=Zero
  Product2 : Product  Inputs=**  RndMeth=Zero
  Real-Imag to Complex : RealImagToComplex
  Saturation : Saturate  UpperLimit=1  LowerLimit=0
  Trigonometric Function : Trigonometry
  Uabc_ref : Outport  VectorParamsAs1DForOutWhenUnconnected=off
  tag scope: m_1_2=global
  wires:
  Constant4/1 -> Add1/4
  wt/1 -> Add1/1
  Product2/1 -> Uabc_ref/1
  Trigonometric Function/1 -> Product2/2
  Saturation/1 -> Product2/1, [m_1_2]
  Add2/1 -> Trigonometric Function/1
  Add1/1 -> Add2/2
  Complex to Magnitude-Angle/2 -> Add2/1
  Product/1 -> Product1/2
  Constant3/1 -> Product/2
  Constant/1 -> Add1/3
  Constant2/1 -> Add1/2
  Demux1/2 -> Real-Imag to Complex/2
  Demux1/1 -> Real-Imag to Complex/1
  Real-Imag to Complex/1 -> Complex to Magnitude-Angle/1
  Gain1/1 -> Product/1
  Product1/1 -> Demux1/1
  VdVq_conv/1 -> Product1/1
  Constant1/1 -> Gain1/1
  Complex to Magnitude-Angle/1 -> Saturation/1

== system Microgrid_w_BESS_Q4_1/VSC Control/VDC Regulator ==
  Vdc_meas : Inport  PortDimensions=1
  Vdc_ref : Inport  Port=2  PortDimensions=1
  PI : slpidlib/PID Controller  Controller=PI  Form=Parallel  TimeDomain=Discrete-time  UseExternalTs=off  SampleTime=Ts  IntegratorMethod=Trapezoidal  FilterMethod=Forward Euler  ControllerParametersSource=internal  P=Kp_VDCreg  I=Ki_VDCreg  UseKiTs=off  D=0  UseExternalDerivativeSource=off  N=100  UseFilter=on  TunerSelectOption=Transfer Function Based (PID Tuner App)  InitialConditionSource=internal  InitialConditionForIntegrator=0  InitialConditionForFilter=0  DifferentiatorICPrevScaledInput=0  ExternalReset=none  TrackingMode=off  Kt=1  LimitOutput=on  SatLimitsSource=internal  UpperSaturationLimit=1.5  LowerSaturationLimit=-1.5  LinearizeAsGain=off  AntiWindupMode=none  Kb=1  LimitIntegrator=off  UpperIntegratorSaturationLimit=inf  LowerIntegratorSaturationLimit=-inf  POutMin=[]  POutMax=[]  IOutMin=[]  IOutMax=[]  DOutMin=[]  DOutMax=[]  NOutMin=[]  NOutMax=[]  SumOutMin=[]  SumOutMax=[]  SaturationOutMin=[]  SaturationOutMax=[]  PParamMin=[]  PParamMax=[]  IParamMin=[]  IParamMax=[]  DParamMin=[]  DParamMax=[]  NParamMin=[]  NParamMax=[]  KbParamMin=[]  KbParamMax=[]  KtParamMin=[]  KtParamMax=[]  KbOutMin=[]  KbOutMax=[]  KtOutMin=[]  KtOutMax=[]  IntegratorOutMin=[]  IntegratorOutMax=[]  FilterOutMin=[]  FilterOutMax=[]  SumI1OutMin=[]  SumI1OutMax=[]  SumI2OutMin=[]  SumI2OutMax=[]  SumI3OutMin=[]  SumI3OutMax=[]  SumI4OutMin=[]  SumI4OutMax=[]  SumDOutMin=[]  SumDOutMax=[]  DifferentiatorOutMin=[]  DifferentiatorOutMax=[]  FilterDiffOutCoefMin=[]  FilterDiffOutCoefMax=[]  ReciprocalOutMin=[]  ReciprocalOutMax=[]  SumDenOutMin=[]  SumDenOutMax=[]  SumNumOutMin=[]  SumNumOutMax=[]  DivideOutMin=[]  DivideOutMax=[]  UdiffTsProdOutMin=[]  UdiffTsProdOutMax=[]  NTsProdOutMin=[]  NTsProdOutMax=[]  UintegralTsProdOutMin=[]  UintegralTsProdOutMax=[]  UngainTsProdOutMin=[]  UngainTsProdOutMax=[]  ClampingZeroOutDataTypeStr=Inherit: Inherit via back propagation  ClampingZeroOutMin=[]  ClampingZeroOutMax=[]  FilterDenConstantOutDataTypeStr=Inherit: Inherit via back propagation  FilterDenConstantOutMin=[]  FilterDenConstantOutMax=[]  PCopyOutDataTypeStr=Inherit: Inherit via back propagation  PCopyOutMin=[]  PCopyOutMax=[]  NCopyOutDataTypeStr=Inherit: Inherit via back propagation  NCopyOutMin=[]  NCopyOutMax=[]  IntegratorContinuousStateAttributes=''  IntegratorStateMustResolveToSignalObject=off  IntegratorRTWStateStorageClass=Auto  FilterContinuousStateAttributes=''  FilterStateMustResolveToSignalObject=off  FilterRTWStateStorageClass=Auto  ParallelPVariant=InternalParameters  IdealPVariant=Disabled  IVariant=InternalParameters  DVariant=Disabled  IntegratorVariant=Discrete  SatVariant=Enabled  AWVariant=Passthrough  PCopyVariant=Disabled  TRVariant=Disabled  FdbkBlocksVariant=Forward  IdealPFdbkVariant=Disabled  SatFdbkVariant=Disabled  DerivativeFilterVariant=Disabled  NVariant=Disabled  NCopyVariant=Disabled_SignalSpec  FilterICVariant=Disabled  IntegratorICVariant=InternalICs  ExternalResetVariant=Disabled  TRSumVariant=Passthrough  SumFdbkVariant=Disabled  SumVariant=Sum_PI  TsampFilterVariant=InternalTs  TsampNgainVariant=Passthrough  TsampIntegralVariant=Disabled_SignalSpec  ExternalSaturationOutDataTypeStr=Inherit: Same as second input  DerivativeSourceVariant=Disabled  PreIntVariant=InternalPreInt
  Rtot_pu3 : Gain  Gain=1/Vnom_dc  SaturateOnIntegerOverflow=on  OutDataTypeStr=Inherit: Same as input  ParamDataTypeStr=Inherit: Same as input
  Sum : Sum  Inputs=|+-
  Id_ref : Outport  SampleTime=Ts  InitialOutput=0  VectorParamsAs1DForOutWhenUnconnected=off
  tag scope: Id_ref_2=global, Vdc_ref_2=global
  wires:
  Rtot_pu3/1 -> PI/1
  Vdc_ref/1 -> [Vdc_ref_2], Sum/2
  Vdc_meas/1 -> Sum/1
  Sum/1 -> Rtot_pu3/1
  PI/1 -> [Id_ref_2], Id_ref/1

== matlab function Microgrid_w_BESS_Q4_1/Scopes/SoC/MATLAB Function1 ==
  settings: updateMethod=DISCRETE
  data: I_batt input; SoC output; V_batt input; initial_SOC input; Q_nom input; time_scale input; Ts input
function SoC = soc_estimation_with_voltage(I_batt, V_batt, initial_SOC, Q_nom, time_scale, Ts)
%#codegen
% Persistent integrator state
persistent integral_charge SoC_coulomb_state
if isempty(integral_charge)
    integral_charge = 0;
    SoC_coulomb_state = initial_SOC;
end

% Time-scaled charge integration (Ah)
delta_charge = (I_batt * Ts) / 3600; % Positive I_batt means charging
integral_charge = integral_charge + delta_charge * time_scale;

% Update Coulomb-based SoC cumulatively
SoC_coulomb_state = SoC_coulomb_state + (delta_charge * time_scale) / Q_nom;

% Clamp internal state (to prevent runaway)
SoC_coulomb_state = max(0, min(0.9, SoC_coulomb_state));
SoC_coulomb = SoC_coulomb_state;

% Voltage-based correction
V_corr = V_batt - I_batt * 0.1; % R_int = 0.1 Ohm
V_ocv_base = 380 + 50 * SoC_coulomb - 5 * SoC_coulomb^2;
SoC_voltage = max(0, min(1, (V_corr - 380) / 50));  % Linear approximation

% Weighted average
SoC = 0.98 * SoC_coulomb + 0.02 * SoC_voltage;
SoC = max(0, min(0.9, SoC));

% Debugging
assignin('base', 'integral_charge', integral_charge);
assignin('base', 'delta_charge', delta_charge);
assignin('base', 'I_batt', I_batt);
assignin('base', 'SoC_coulomb', SoC_coulomb);
assignin('base', 'SoC_voltage', SoC_voltage);
assignin('base', 'SoC', SoC);
assignin('base', 'V_batt', V_batt);
assignin('base', 'V_ocv_base', V_ocv_base);
assignin('base', 'V_corr', V_corr);
end

== matlab function Microgrid_w_BESS_Q4_1/Scopes/MATLAB Function ==
  settings: updateMethod=DISCRETE
  data: P_grid input; E_imp output; E_exp output; Tariff input; FiT input; Ts input; Cost output; Revenue output; NetCost output; ScaleFactor input
function [E_imp, E_exp, Cost, Revenue, NetCost] = tariff_calc(P_grid, Tariff, FiT, Ts, ScaleFactor)
% Inputs:
% - P_grid: grid power in Watts (+ for import, - for export)
% - Tariff: import tariff in cent/kWh
% - FiT: feed-in tariff in cent/kWh
% - Ts: Simulink timestep in seconds
% - ScaleFactor: time compression factor (e.g. 86400/4 = 21600)

% Outputs (all time-scaled):
% - E_imp: Imported energy in kWh
% - E_exp: Exported energy in kWh
% - Cost: Import cost in euros
% - Revenue: Export earnings in euros
% - NetCost: Cost - Revenue in euros

persistent e_imp e_exp cost revenue
if isempty(e_imp)
    e_imp = 0; e_exp = 0; cost = 0; revenue = 0;
end

% Convert tariff and FiT from cent to euro
Tariff_eur = Tariff / 100;
FiT_eur = FiT / 100;

% Real-time duration of the current timestep
real_Ts = Ts * ScaleFactor;

% Convert W to kWh: P × real_Ts / 3.6e6
if P_grid > 0
    e_step = P_grid * real_Ts / 3600000;
    e_imp = e_imp + e_step;
    cost = cost + e_step * Tariff_eur;
elseif P_grid < 0
    p_exp = -P_grid;
    e_step = p_exp * real_Ts / 3600000;
    e_exp = e_exp + e_step;
    revenue = revenue + e_step * FiT_eur;
end

E_imp = e_imp;
E_exp = e_exp;
Cost = cost;
Revenue = revenue;
NetCost = cost - revenue;

end

== matlab function Microgrid_w_BESS_Q4_1/BESS/BATT chg-dshg logic1/MATLAB Function ==
  data: price input; mode output
function mode = tariff_dynamic_discharge(price)
%#codegen
% BESS discharges when price ≥ 20, charges when price < 20.
% Initially discharges because battery is full.

    threshold = 20;

    if price >= threshold
        mode = 0.0;  % Discharging
    else
        mode = 1.0;  % Charging
    end
end

== matlab function Microgrid_w_BESS_Q4_1/Scopes/MATLAB Function1 ==
  settings: updateMethod=DISCRETE
  data: P_watt input; E_kWh output; Tariff_cent input; FixedTariff_cent input; Ts input; ScaleFactor input; Cost_dynamic_eur output; Cost_fixed_eur output; Cost_diff output
function [E_kWh, Cost_dynamic_eur, Cost_fixed_eur, Cost_diff] = correct_tariff(P_watt, Tariff_cent, FixedTariff_cent, Ts, ScaleFactor)

persistent E_acc Cost_dynamic_acc Cost_fixed_acc
if isempty(E_acc)
    E_acc = 0;
    Cost_dynamic_acc = 0;
    Cost_fixed_acc = 0;
end

% Convert power to energy in kWh (scaled time)
E_step = (P_watt * Ts * ScaleFactor) / 3600000;  % W * s / 3.6e6 = kWh

% Convert tariffs from cent/kWh to €/kWh
Tariff_dynamic_eur = Tariff_cent / 100;
Tariff_fixed_eur   = FixedTariff_cent / 100;

% Cost per step
Cost_step_dynamic = E_step * Tariff_dynamic_eur;
Cost_step_fixed   = E_step * Tariff_fixed_eur;

% Accumulate
E_acc = E_acc + E_step;
Cost_dynamic_acc = Cost_dynamic_acc + Cost_step_dynamic;
Cost_fixed_acc   = Cost_fixed_acc + Cost_step_fixed;

% Outputs
E_kWh            = E_acc;
Cost_dynamic_eur = Cost_dynamic_acc;
Cost_fixed_eur   = Cost_fixed_acc;
Cost_diff        = Cost_fixed_acc - Cost_dynamic_acc;

end

== matlab function Microgrid_w_BESS_Q4_1/Scopes/MATLAB Function2 ==
  settings: updateMethod=DISCRETE
  data: P_grid input; E_exp output; FiT input; Ts input; Revenue output; ScaleFactor input
function [E_exp, Revenue] = full_fit_calc(P_grid, FiT, Ts, ScaleFactor)
% Calculates energy exported and revenue from feed-in tariff (FiT)
%
% Inputs:
% - P_grid: grid power in Watts (negative for export)
% - FiT: feed-in tariff in cent/kWh
% - Ts: Simulink timestep in seconds
% - ScaleFactor: time compression factor (e.g. 86400/4 = 21600)
%
% Outputs (time-accumulated):
% - E_exp: Exported energy in kWh
% - Revenue: Export earnings in euros

persistent e_exp revenue
if isempty(e_exp)
    e_exp = 0;
    revenue = 0;
end

% Convert FiT from cent to euro
FiT_eur = FiT / 100;

% Real-time duration of the current timestep
real_Ts = Ts * ScaleFactor;

% Convert power to energy in kWh
if P_grid < 0
    p_exp = -P_grid;  % export power (make positive)
    e_step = p_exp * real_Ts / 3600000;  % W·s → kWh
    e_exp = e_exp + e_step;
    revenue = revenue + e_step * FiT_eur;
end

% Outputs
E_exp = e_exp;
Revenue = revenue;

end

== matlab function Microgrid_w_BESS_Q4_1/Scopes/MATLAB Function3 ==
  settings: updateMethod=DISCRETE
  data: P_grid input; E_exp output; FiT input; Ts input; Revenue output; ScaleFactor input
function [E_exp, Revenue] = full_fit_calc(P_grid, FiT, Ts, ScaleFactor)
% Calculates energy exported and revenue from feed-in tariff (FiT)
%
% Inputs:
% - P_grid: grid power in Watts (negative for export)
% - FiT: feed-in tariff in cent/kWh
% - Ts: Simulink timestep in seconds
% - ScaleFactor: time compression factor (e.g. 86400/4 = 21600)
%
% Outputs (time-accumulated):
% - E_exp: Exported energy in kWh
% - Revenue: Export earnings in euros

persistent e_exp revenue
if isempty(e_exp)
    e_exp = 0;
    revenue = 0;
end

% Convert FiT from cent to euro
FiT_eur = FiT / 100;

% Real-time duration of the current timestep
real_Ts = Ts * ScaleFactor;

% Convert power to energy in kWh
if P_grid < 0
    p_exp = -P_grid;  % export power (make positive)
    e_step = p_exp * real_Ts / 3600000;  % W·s → kWh
    e_exp = e_exp + e_step;
    revenue = revenue + e_step * FiT_eur;
end

% Outputs
E_exp = e_exp;
Revenue = revenue;

end
